simulink model "ExoskeletonFuzzyPID"  (R2016a)
settings: Solver=VariableStepAuto  StartTime=0.0  StopTime=10.0  RelTol=1e-3
values from neighbouring files (symbols this model uses):
  Bm = 0.002953    [April2code.mat]    (also in April6code.mat)
  Kd = 0.45    [April2code.mat]    (also in April6code.mat = 0.7)
  Kp = 5    [April2code.mat]    (also in April6code.mat = 8)
  La = 0.1215    [April2code.mat]    (also in April6code.mat)
  Ra = 11.2    [April2code.mat]    (also in April6code.mat)
undefined symbols (not defined in the file or in its folder): flux_e, J
libraries: fuzblock x1
settings Model: Creator=Dheeraj Singh  LastModifiedBy=Dheeraj Singh

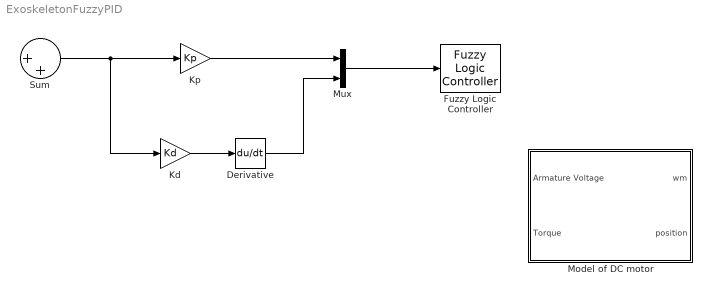
== system ExoskeletonFuzzyPID ==
  Derivative : Derivative
  Fuzzy Logic Controller : fuzblock/Fuzzy Logic  Controller  fis=ExoskeletonFuzzy.fis
  Kd : Gain  Gain=Kd
  Kp : Gain  Gain=Kp
  Model of DC motor : Subsystem
  Mux : Mux  Inputs=2
  Sum : Sum  Inputs=|++
  wires:
  Sum/1 -> Kd/1, Kp/1
  Kd/1 -> Derivative/1
  Kp/1 -> Mux/1
  Derivative/1 -> Mux/2
  Mux/1 -> Fuzzy Logic Controller/1

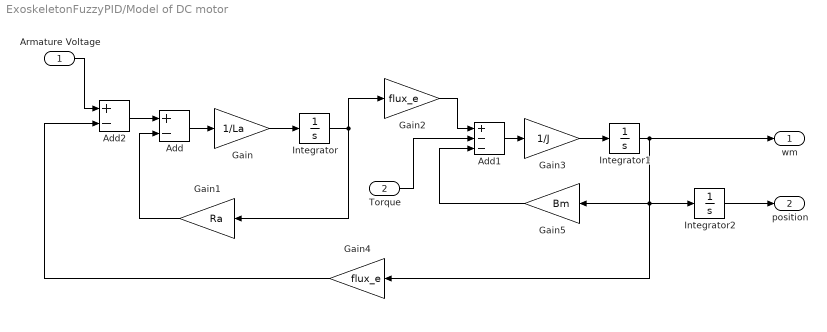
== system ExoskeletonFuzzyPID/Model of DC motor ==
  Armature Voltage : Inport
  Torque : Inport  Port=2
  Add : Sum  Inputs=+-
  Add1 : Sum  Inputs=+--
  Add2 : Sum  Inputs=+-
  Gain : Gain  Gain=1/La
  Gain1 : Gain  Gain=Ra
  Gain2 : Gain  Gain=flux_e
  Gain3 : Gain  Gain=1/J
  Gain4 : Gain  Gain=flux_e
  Gain5 : Gain  Gain=Bm
  Integrator : Integrator
  Integrator1 : Integrator
  Integrator2 : Integrator
  wm : Outport
  position : Outport  Port=2
  wires:
  Gain/1 -> Integrator/1
  Integrator/1 -> Gain1/1, Gain2/1
  Add/1 -> Gain/1
  Gain1/1 -> Add/2
  Gain2/1 -> Add1/1
  Add1/1 -> Gain3/1
  Gain3/1 -> Integrator1/1
  Add2/1 -> Add/1
  Gain4/1 -> Add2/2
  Integrator1/1 -> wm/1, Gain4/1, Integrator2/1, Gain5/1
  Torque/1 -> Add1/2
  Armature Voltage/1 -> Add2/1
  Gain5/1 -> Add1/3
  Integrator2/1 -> position/1
